simulink model "piezo"  (R2020b)
settings: Solver=VariableStepAuto  StartTime=0.0  StopTime=10.0  FixedStep=1e-6  RelTol=1e-3
libraries: slident x1
settings Model: Creator=Salvatore  LastModifiedBy=Salvatore

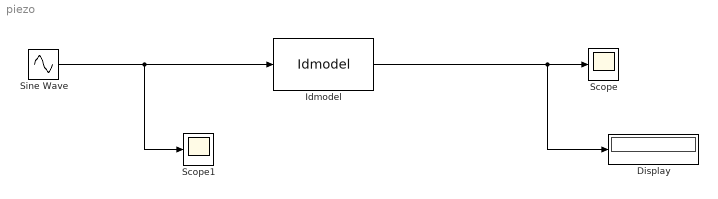
== system piezo ==
  Display : Display
  Idmodel : slident/Models/Idmodel  sys=n4s3  IC=0  noi=on  seed=[]
      settings: SourceProductBaseCode=ID
  Scope : Scope
  Scope1 : Scope
  Sine Wave : Sin  Frequency=2*pi*10e3  SampleTime=0
  wires:
  Idmodel/1 -> Display/1, Scope/1
  Sine Wave/1 -> Scope1/1, Idmodel/1
